simulink model "codegen_02"  (R2013b)
settings: Solver=FixedStepDiscrete  StartTime=0.0  StopTime=10.0  RelTol=1e-3
values from neighbouring files (symbols this model uses):
  k = mpt.Parameter    [chap17_02_83_script.m]    (also in codegen_02s.m)
settings Model: Creator=Administrator  LastModifiedBy=Administrator
settings OptimizationCC: InlineParams=on  EnhancedBackFolding=on  OptimizeModelRefInitCode=on  LifeSpan=1
settings RTWCC: SystemTargetFile=ert.tlc  GenCodeOnly=on  TemplateMakefile=ert_default_tmf  Description=Embedded Coder  GenerateReport=on  ProcessScript=ert_make_rtw_hook  IncludeHyperlinkInReport=on  LaunchReport=on
settings CodeAppCC: IgnoreCustomStorageClasses=off
settings ERTTargetCC: CodeReplacementLibrary=ANSI_C  GenerateSampleERTMain=on  ERTCustomFileTemplate=example_file_process.tlc

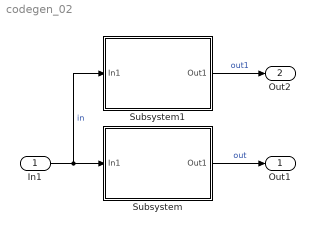
== system codegen_02 ==
  In1 : Inport
  Subsystem : Subsystem  TreatAsAtomicUnit=on  RTWFcnName=gain_fun  RTWFileName=subsys_fun
      settings: RTWFcnNameOpts=User specified  RTWFileNameOpts=User specified  FunctionInterfaceSpec=Allow arguments  FunctionWithSeparateData=on
  Subsystem1 : Subsystem  TreatAsAtomicUnit=on  RTWFcnName=gain_fun  RTWFileName=subsys_fun
      settings: RTWFcnNameOpts=User specified  RTWFileNameOpts=User specified  FunctionInterfaceSpec=Allow arguments  FunctionWithSeparateData=on
  Out1 : Outport
  Out2 : Outport  Port=2
  wires:
  In1/1 -> Subsystem1/1(In1), Subsystem/1(In1)  "in"
  Subsystem/1(Out1) -> Out1/1  "out"
  Subsystem1/1(Out1) -> Out2/1  "out1"

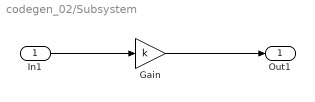
== system codegen_02/Subsystem ==
  In1 : Inport
  Gain : Gain  Gain=k
  Out1 : Outport
  wires:
  In1/1 -> Gain/1
  Gain/1 -> Out1/1

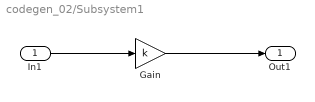
== system codegen_02/Subsystem1 ==
  In1 : Inport
  Gain : Gain  Gain=k
  Out1 : Outport
  wires:
  In1/1 -> Gain/1
  Gain/1 -> Out1/1
